simulink model "simulink_model_sil"  (R2022b)
settings: Solver=FixedStepDiscrete  StartTime=0.0  StopTime=10  FixedStep=0.2  RelTol=1e-3
libraries: simulink x2, pil_lib x1
settings Model: Creator=ahmed  LastModifiedBy=ahmed
settings SolverCC: AlgebraicLoopSolver=TrustRegion
settings DataIOCC: ReturnWorkspaceOutputs=off
settings OptimizationCC: DefaultParameterBehavior=Inlined  UseDivisionForNetSlopeComputation=on  GainParamInheritBuiltInType=on  UseFloatMulNetSlope=on  InlineInvariantSignals=on  PassReuseOutputArgsAs=Individual arguments  ZeroExternalMemoryAtStartup=off  ZeroInternalMemoryAtStartup=off  NoFixptDivByZeroProtection=on  EfficientFloat2IntCast=on  LifeSpan=1  OptimizeBlockOrder=speed  DifferentSizesBufferReuse=on  EfficientTunableParamExpr=on
settings DebuggingCC: ParameterTunabilityLossMsg=error  UnconnectedInputMsg=warning  UnconnectedOutputMsg=warning  UnconnectedLineMsg=warning  SFMachineParentedDataDiag=warning  ArithmeticOperatorsInVariantConditions=warning
settings HardwareCC: ProdBitPerInt=16  ProdBitPerPointer=16  ProdBitPerSizeT=16  ProdBitPerPtrDiffT=16  ProdLargestAtomicFloat=None  ProdWordSize=8  ProdLongLongMode=on  ProdHWDeviceType=Atmel->AVR  TargetBitPerPointer=64  TargetBitPerSizeT=64  TargetBitPerPtrDiffT=64  TargetLongLongMode=on  TargetIntDivRoundTo=Zero  TargetEndianess=LittleEndian  TargetWordSize=64  TargetHWDeviceType=Generic->MATLAB Host Computer  ProdEqTarget=off
settings ModelReferenceCC: EnableRefExpFcnMdlSchedulingChecks=on
settings SFSimCC: SimUseLocalCustomCode=off  MATLABDynamicMemAlloc=off  CustomCodeUndefinedFunction=UseInterfaceOnly
settings RTWCC: Description=Embedded Coder  SystemTargetFile=ert.tlc  TemplateMakefile=ert_default_tmf  GenerateReport=on  RTWUseLocalCustomCode=off  IncludeHyperlinkInReport=on  LaunchReport=on  GenerateTraceInfo=on  GenerateTraceReport=on  GenerateTraceReportSl=on  GenerateTraceReportSf=on  GenerateTraceReportEml=on  GenerateCodeMetricsReport=on
settings CodeAppCC: ForceParamTrailComments=on  IgnoreCustomStorageClasses=off  OperatorAnnotations=on  SimulinkDataObjDesc=on  SFDataObjDesc=on  CustomSymbolStrGlobalVar=rt$N$M  CustomSymbolStrType=$N$M  CustomSymbolStrFcn=$N$M$F  CustomSymbolStrMacro=$N$M  InsertBlockDesc=on
settings ERTTargetCC: TargetLangStandard=C99 (ISO)  GenerateSampleERTMain=on  IncludeMdlTerminateFcn=off  CombineSignalStateStructs=on  SuppressErrorStatus=on  SupportAbsoluteTime=off  SupportComplex=off  InlinedParameterPlacement=NonHierarchical  ERTCustomFileTemplate=example_file_process.tlc  ERTFilePackagingFormat=CompactWithDataFile

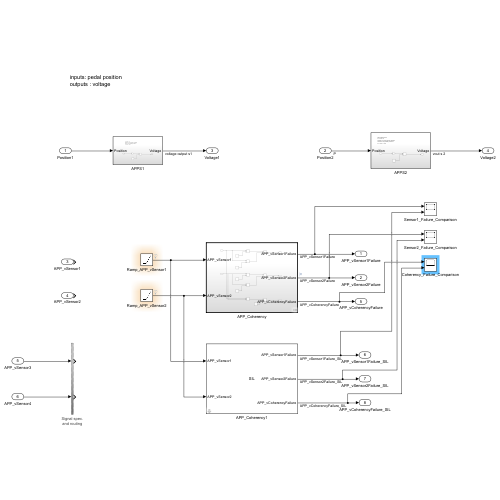
[thumbnail: Simulink's stored preview of the top-level diagram]
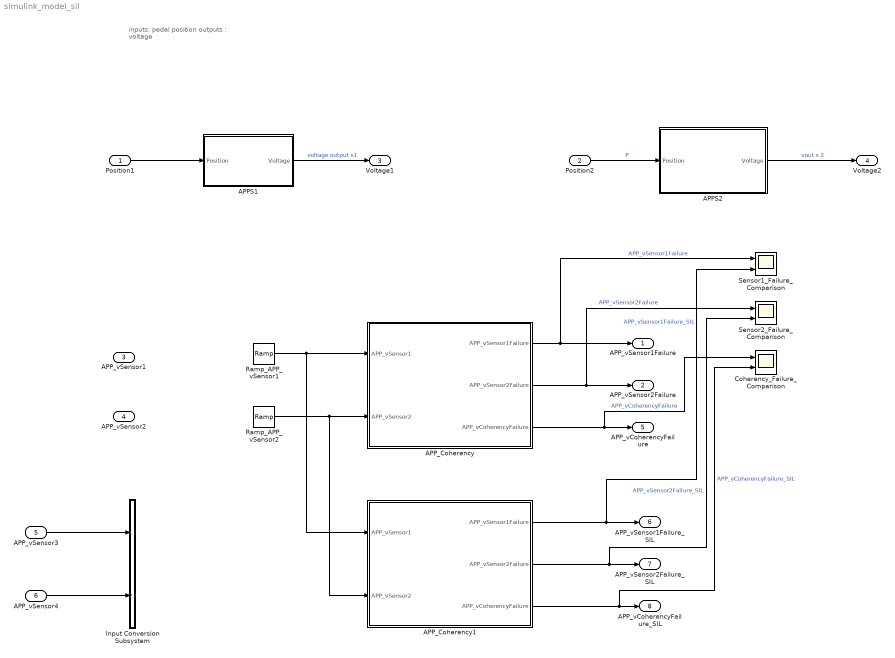
== system simulink_model_sil ==
  note: inputs: pedal position
      | outputs : voltage
  Position1 : Inport
  Position2 : Inport  Port=2
  APP_vSensor1 : Inport  Port=3
  APP_vSensor2 : Inport  Port=4
  APP_vSensor3 : Inport  Port=5  OutDataTypeStr=double  PortDimensions=[1]  SampleTime=0.2
  APP_vSensor4 : Inport  Port=6  OutDataTypeStr=double  PortDimensions=[1]  SampleTime=0.2
  APPS1 : Subsystem
  APPS2 : Subsystem
  APP_Coherency : Subsystem  TreatAsAtomicUnit=on
  APP_Coherency1 : Subsystem  Tag=__SL_testing_harness_stub_  DialogController=pil_create_dialog  LoadFcn=|
      | try
      |    if ~strcmp(rtw.pil.getPILVersion, '9.13 (R2022b)_15')
      |       set_param(gcb, 'DialogController', '');
      |       set_param(gcb, 'DialogControllerArgs', '');
      |    end
      | catch e
      |       set_param(gcb, 'DialogController', '');
      |       set_param(gcb, 'DialogControllerArgs', '');
      | end
      mask help: PIL:pil:XILBlockMaskDesc
      mask Display: disp('SIL');
  Coherency_Failure_Comparison : Scope  NumInputPorts=2
  Input Conversion Subsystem : Subsystem  Tag=__SLT_ICS__  Description=|
      | Signal spec.
      | and routing
      settings: AttributesFormatString=%<Description>
  Ramp_APP_vSensor1 : simulink/Sources/Ramp  slope=0.45  start=0  InitialOutput=0
  Ramp_APP_vSensor2 : simulink/Sources/Ramp  slope=-0.4  start=0  InitialOutput=4.5
  Sensor1_Failure_Comparison : Scope  NumInputPorts=2
  Sensor2_Failure_Comparison : Scope  NumInputPorts=2
  APP_vSensor1Failure : Outport  VectorParamsAs1DForOutWhenUnconnected=off
  APP_vSensor2Failure : Outport  Port=2  VectorParamsAs1DForOutWhenUnconnected=off
  Voltage1 : Outport  Port=3  VectorParamsAs1DForOutWhenUnconnected=off
  Voltage2 : Outport  Port=4  VectorParamsAs1DForOutWhenUnconnected=off
  APP_vCoherencyFailure : Outport  Port=5  VectorParamsAs1DForOutWhenUnconnected=off
  APP_vSensor1Failure_SIL : Outport  Port=6
  APP_vSensor2Failure_SIL : Outport  Port=7
  APP_vCoherencyFailure_SIL : Outport  Port=8
  wires:
  APPS1/1(Voltage) -> Voltage1/1  "voltage output s1"
  APPS2/1(Voltage) -> Voltage2/1  "vout s 2"
  APP_Coherency/1(APP_vSensor1Failure) -> APP_vSensor1Failure/1, Sensor1_Failure_Comparison/1  "APP_vSensor1Failure"
  APP_Coherency/2(APP_vSensor2Failure) -> APP_vSensor2Failure/1, Sensor2_Failure_Comparison/1  "APP_vSensor2Failure"
  APP_Coherency/3(APP_vCoherencyFailure) -> Coherency_Failure_Comparison/1, APP_vCoherencyFailure/1  "APP_vCoherencyFailure"
  Position1/1 -> APPS1/1(Position)
  Position2/1 -> APPS2/1(Position)  "P"
  APP_vSensor4/1 -> Input Conversion Subsystem/2(Inport_2)
  APP_vSensor3/1 -> Input Conversion Subsystem/1(Inport_1)
  APP_Coherency1/3(APP_vCoherencyFailure) -> Coherency_Failure_Comparison/2, APP_vCoherencyFailure_SIL/1  "APP_vCoherencyFailure_SIL"
  APP_Coherency1/2(APP_vSensor2Failure) -> Sensor2_Failure_Comparison/2, APP_vSensor2Failure_SIL/1  "APP_vSensor2Failure_SIL"
  APP_Coherency1/1(APP_vSensor1Failure) -> Sensor1_Failure_Comparison/2, APP_vSensor1Failure_SIL/1  "APP_vSensor1Failure_SIL"
  Ramp_APP_vSensor1/1 -> APP_Coherency/1(APP_vSensor1), APP_Coherency1/1(APP_vSensor1)
  Ramp_APP_vSensor2/1 -> APP_Coherency/2(APP_vSensor2), APP_Coherency1/2(APP_vSensor2)

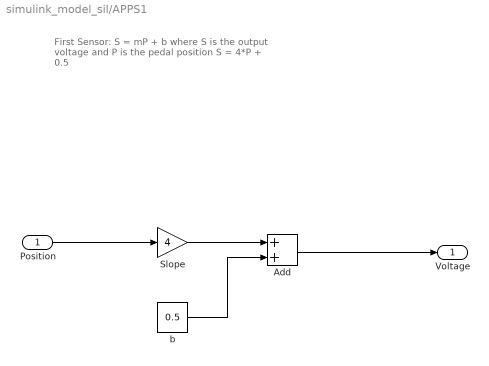
== system simulink_model_sil/APPS1 ==
  note: First Sensor:
      | S = mP + b
      | where S is the output voltage
      | and P is the pedal position
      | S = 4*P + 0.5
  Position : Inport
  Add : Sum
  Slope : Gain  Gain=4
  "b " : Constant  Value=0.5
  Voltage : Outport  VectorParamsAs1DForOutWhenUnconnected=off
  wires:
  Slope/1 -> Add/1
  "b "/1 -> Add/2
  Add/1 -> Voltage/1
  Position/1 -> Slope/1

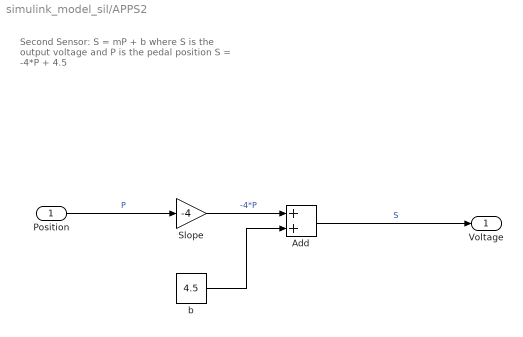
== system simulink_model_sil/APPS2 ==
  note: Second Sensor:
      | S = mP + b
      | where S is the output voltage
      | and P is the pedal position
      | S = -4*P + 4.5
  Position : Inport
  Add : Sum
  Slope : Gain  Gain=-4
  "b " : Constant  Value=4.5
  Voltage : Outport  VectorParamsAs1DForOutWhenUnconnected=off
  wires:
  Slope/1 -> Add/1  "-4*P"
  Add/1 -> Voltage/1  "S"
  Position/1 -> Slope/1  "P"
  "b "/1 -> Add/2

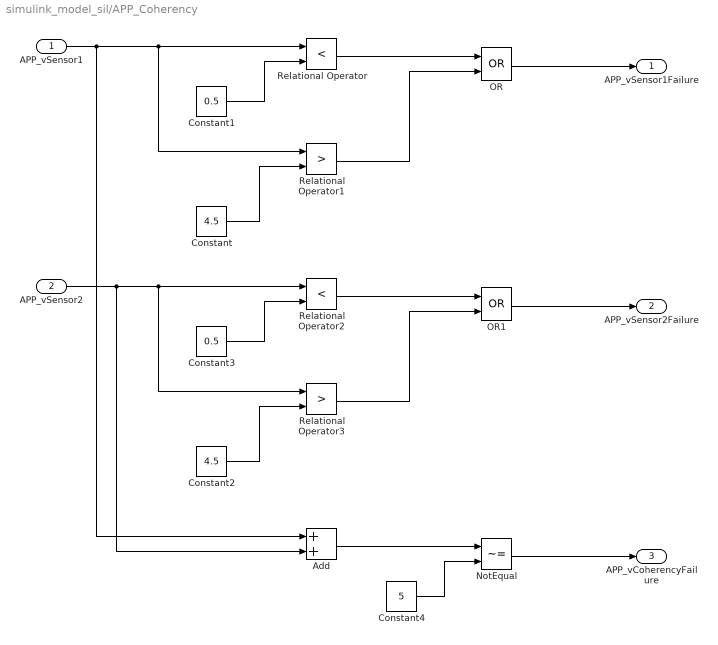
== system simulink_model_sil/APP_Coherency ==
  APP_vSensor1 : Inport
  APP_vSensor2 : Inport  Port=2
  Add : Sum
  Constant : Constant  Value=4.5
  Constant1 : Constant  Value=0.5
  Constant2 : Constant  Value=4.5
  Constant3 : Constant  Value=0.5
  Constant4 : Constant  Value=5
  NotEqual : RelationalOperator  Operator=~=  OutDataTypeStr=boolean  RndMeth=Simplest  InputSameDT=off
  OR : Logic  Operator=OR  AllPortsSameDT=off  OutDataTypeStr=boolean
  OR1 : Logic  Operator=OR  AllPortsSameDT=off  OutDataTypeStr=boolean
  Relational Operator : RelationalOperator  Operator=<  OutDataTypeStr=boolean  RndMeth=Simplest  InputSameDT=off
  Relational Operator1 : RelationalOperator  Operator=>  OutDataTypeStr=boolean  RndMeth=Simplest  InputSameDT=off
  Relational Operator2 : RelationalOperator  Operator=<  OutDataTypeStr=boolean  RndMeth=Simplest  InputSameDT=off
  Relational Operator3 : RelationalOperator  Operator=>  OutDataTypeStr=boolean  RndMeth=Simplest  InputSameDT=off
  APP_vSensor1Failure : Outport  VectorParamsAs1DForOutWhenUnconnected=off
  APP_vSensor2Failure : Outport  Port=2  VectorParamsAs1DForOutWhenUnconnected=off
  APP_vCoherencyFailure : Outport  Port=3  VectorParamsAs1DForOutWhenUnconnected=off
  wires:
  APP_vSensor1/1 -> Add/1, Relational Operator/1, Relational Operator1/1
  Constant1/1 -> Relational Operator/2
  Relational Operator/1 -> OR/1
  Constant/1 -> Relational Operator1/2
  Relational Operator1/1 -> OR/2
  OR/1 -> APP_vSensor1Failure/1
  OR1/1 -> APP_vSensor2Failure/1
  APP_vSensor2/1 -> Add/2, Relational Operator2/1, Relational Operator3/1
  Constant3/1 -> Relational Operator2/2
  Constant2/1 -> Relational Operator3/2
  Relational Operator3/1 -> OR1/2
  Relational Operator2/1 -> OR1/1
  Add/1 -> NotEqual/1
  Constant4/1 -> NotEqual/2
  NotEqual/1 -> APP_vCoherencyFailure/1

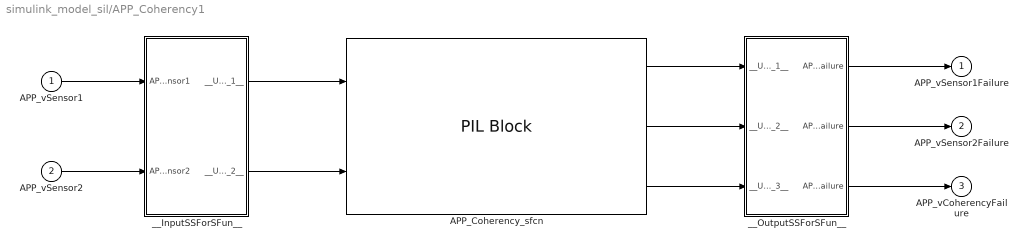
== system simulink_model_sil/APP_Coherency1 ==
  APP_vSensor1 : Inport
  APP_vSensor2 : Inport  Port=2
  APP_Coherency_sfcn : pil_lib/PIL Block  SimulationMode=SIL  IsTopModelPIL=off  CodeDir=APP_Coherency_ert_rtw  AnchorDir=D:\yarab  ConfigName=Software-in-the-Loop (SIL)  XrelIsTopModelCode=on  XrelIsReusable=off  XrelDWorkNames={}  XrelDWorkTypes={}  XrelModelArgVals={}  XrelOrderedParamNames={}
  __InputSSForSFun__ : Subsystem
  __OutputSSForSFun__ : Subsystem
  APP_vSensor1Failure : Outport  VectorParamsAs1DForOutWhenUnconnected=off
  APP_vSensor2Failure : Outport  Port=2  VectorParamsAs1DForOutWhenUnconnected=off
  APP_vCoherencyFailure : Outport  Port=3  VectorParamsAs1DForOutWhenUnconnected=off
  wires:
  __OutputSSForSFun__/3(APP_vCoherencyFailure) -> APP_vCoherencyFailure/1
  __OutputSSForSFun__/2(APP_vSensor2Failure) -> APP_vSensor2Failure/1
  __OutputSSForSFun__/1(APP_vSensor1Failure) -> APP_vSensor1Failure/1
  APP_Coherency_sfcn/3 -> __OutputSSForSFun__/3(__UniqueInportName__3__)
  APP_Coherency_sfcn/2 -> __OutputSSForSFun__/2(__UniqueInportName__2__)
  APP_Coherency_sfcn/1 -> __OutputSSForSFun__/1(__UniqueInportName__1__)
  __InputSSForSFun__/2(__UniqueOutportName__2__) -> APP_Coherency_sfcn/2
  __InputSSForSFun__/1(__UniqueOutportName__1__) -> APP_Coherency_sfcn/1
  APP_vSensor2/1 -> __InputSSForSFun__/2(APP_vSensor2)
  APP_vSensor1/1 -> __InputSSForSFun__/1(APP_vSensor1)

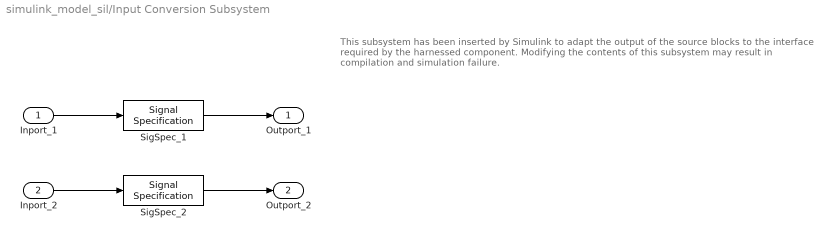
== system simulink_model_sil/Input Conversion Subsystem ==
  note: This subsystem has been inserted by Simulink to adapt the output of the source blocks to the interface required by the harnessed component.
      |  Modifying the contents of this subsystem may result in compilation and simulation failure.
  Inport_1 : Inport
  Inport_2 : Inport  Port=2
  SigSpec_1 : SignalSpecification  OutDataTypeStr=double  Dimensions=[1]  SampleTime=0.2
  SigSpec_2 : SignalSpecification  OutDataTypeStr=double  Dimensions=[1]  SampleTime=0.2
  Outport_1 : Outport
  Outport_2 : Outport  Port=2
  wires:
  SigSpec_1/1 -> Outport_1/1
  Inport_1/1 -> SigSpec_1/1
  SigSpec_2/1 -> Outport_2/1
  Inport_2/1 -> SigSpec_2/1

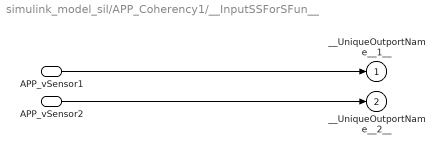
== system simulink_model_sil/APP_Coherency1/__InputSSForSFun__ ==
  APP_vSensor1 : Inport
  APP_vSensor2 : Inport  Port=2
  __UniqueOutportName__1__ : Outport
  __UniqueOutportName__2__ : Outport  Port=2
  wires:
  APP_vSensor2/1 -> __UniqueOutportName__2__/1
  APP_vSensor1/1 -> __UniqueOutportName__1__/1

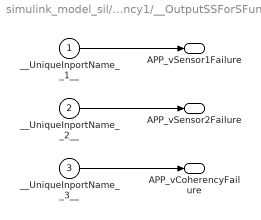
== system simulink_model_sil/APP_Coherency1/__OutputSSForSFun__ ==
  __UniqueInportName__1__ : Inport
  __UniqueInportName__2__ : Inport  Port=2
  __UniqueInportName__3__ : Inport  Port=3
  APP_vSensor1Failure : Outport  VectorParamsAs1DForOutWhenUnconnected=off
  APP_vSensor2Failure : Outport  Port=2  VectorParamsAs1DForOutWhenUnconnected=off
  APP_vCoherencyFailure : Outport  Port=3  VectorParamsAs1DForOutWhenUnconnected=off
  wires:
  __UniqueInportName__3__/1 -> APP_vCoherencyFailure/1
  __UniqueInportName__2__/1 -> APP_vSensor2Failure/1
  __UniqueInportName__1__/1 -> APP_vSensor1Failure/1
